simulink model "Multiplier"  (R2019b)
settings: Solver=VariableStepAuto  StartTime=0.0  StopTime=10.0  RelTol=1e-3
libraries: hdlsllib x17
(part 2 of 3)

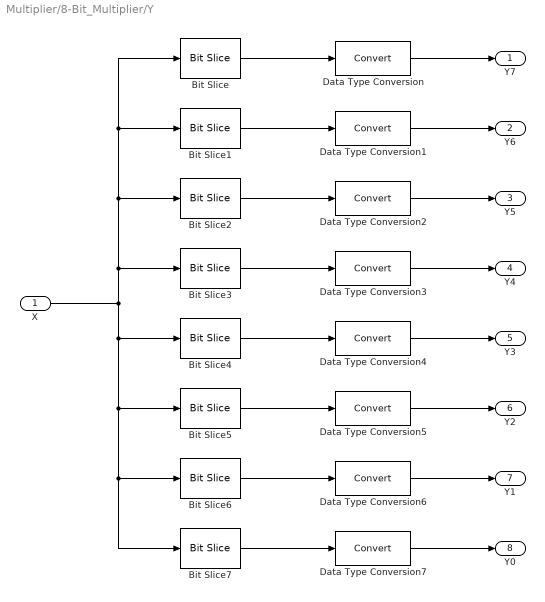
== system Multiplier/8-Bit_Multiplier/Y ==
  X : Inport  OutDataTypeStr=uint8  SampleTime=1
  Bit Slice : hdlsllib/Logic and Bit Operations/Bit Slice  lidx=7  ridx=7
      settings: SourceProductName=Simulink  SourceProductBaseCode=SL
  Bit Slice1 : hdlsllib/Logic and Bit Operations/Bit Slice  lidx=6  ridx=6
      settings: SourceProductName=Simulink  SourceProductBaseCode=SL
  Bit Slice2 : hdlsllib/Logic and Bit Operations/Bit Slice  lidx=5  ridx=5
      settings: SourceProductName=Simulink  SourceProductBaseCode=SL
  Bit Slice3 : hdlsllib/Logic and Bit Operations/Bit Slice  lidx=4  ridx=4
      settings: SourceProductName=Simulink  SourceProductBaseCode=SL
  Bit Slice4 : hdlsllib/Logic and Bit Operations/Bit Slice  lidx=3  ridx=3
      settings: SourceProductName=Simulink  SourceProductBaseCode=SL
  Bit Slice5 : hdlsllib/Logic and Bit Operations/Bit Slice  lidx=2  ridx=2
      settings: SourceProductName=Simulink  SourceProductBaseCode=SL
  Bit Slice6 : hdlsllib/Logic and Bit Operations/Bit Slice  lidx=1  ridx=1
      settings: SourceProductName=Simulink  SourceProductBaseCode=SL
  Bit Slice7 : hdlsllib/Logic and Bit Operations/Bit Slice  lidx=0  ridx=0
      settings: SourceProductName=Simulink  SourceProductBaseCode=SL
  Data Type Conversion{,1..7} (8 alike) : DataTypeConversion
  Y7 : Outport
  Y6 : Outport  Port=2
  Y5 : Outport  Port=3
  Y4 : Outport  Port=4
  Y3 : Outport  Port=5
  Y2 : Outport  Port=6
  Y1 : Outport  Port=7
  Y0 : Outport  Port=8
  wires:
  Bit Slice6/1 -> Data Type Conversion6/1
  X/1 -> Bit Slice3/1, Bit Slice2/1, Bit Slice1/1, Bit Slice/1, Bit Slice4/1, Bit Slice5/1, Bit Slice6/1, Bit Slice7/1
  Bit Slice/1 -> Data Type Conversion/1
  Bit Slice7/1 -> Data Type Conversion7/1
  Bit Slice4/1 -> Data Type Conversion4/1
  Bit Slice1/1 -> Data Type Conversion1/1
  Bit Slice3/1 -> Data Type Conversion3/1
  Data Type Conversion1/1 -> Y6/1
  Data Type Conversion7/1 -> Y0/1
  Data Type Conversion5/1 -> Y2/1
  Data Type Conversion3/1 -> Y4/1
  Data Type Conversion4/1 -> Y3/1
  Bit Slice2/1 -> Data Type Conversion2/1
  Bit Slice5/1 -> Data Type Conversion5/1
  Data Type Conversion6/1 -> Y1/1
  Data Type Conversion/1 -> Y7/1
  Data Type Conversion2/1 -> Y5/1

== system Multiplier/8-Bit_Multiplier/Full adder1/Half adder1 ==
  In1 : Inport  OutDataTypeStr=boolean
  In2 : Inport  Port=2  OutDataTypeStr=boolean
  Logical Operator : Logic  AllPortsSameDT=off  OutDataTypeStr=boolean
  Logical Operator1 : Logic  Operator=XOR  AllPortsSameDT=off  OutDataTypeStr=boolean
  Out1 : Outport
  Out2 : Outport  Port=2
  wires:
  In2/1 -> Logical Operator/2, Logical Operator1/2
  In1/1 -> Logical Operator/1, Logical Operator1/1
  Logical Operator1/1 -> Out1/1
  Logical Operator/1 -> Out2/1

== system Multiplier/8-Bit_Multiplier/Full adder1/Half adder2 ==
  In1 : Inport  OutDataTypeStr=boolean
  In2 : Inport  Port=2  OutDataTypeStr=boolean
  Logical Operator : Logic  AllPortsSameDT=off  OutDataTypeStr=boolean
  Logical Operator1 : Logic  Operator=XOR  AllPortsSameDT=off  OutDataTypeStr=boolean
  Out1 : Outport
  Out2 : Outport  Port=2
  wires:
  In2/1 -> Logical Operator/2, Logical Operator1/2
  In1/1 -> Logical Operator/1, Logical Operator1/1
  Logical Operator1/1 -> Out1/1
  Logical Operator/1 -> Out2/1

== system Multiplier/8-Bit_Multiplier/Full adder10/Half adder1 ==
  In1 : Inport  OutDataTypeStr=boolean
  In2 : Inport  Port=2  OutDataTypeStr=boolean
  Logical Operator : Logic  AllPortsSameDT=off  OutDataTypeStr=boolean
  Logical Operator1 : Logic  Operator=XOR  AllPortsSameDT=off  OutDataTypeStr=boolean
  Out1 : Outport
  Out2 : Outport  Port=2
  wires:
  In2/1 -> Logical Operator/2, Logical Operator1/2
  In1/1 -> Logical Operator/1, Logical Operator1/1
  Logical Operator1/1 -> Out1/1
  Logical Operator/1 -> Out2/1

== system Multiplier/8-Bit_Multiplier/Full adder10/Half adder2 ==
  In1 : Inport  OutDataTypeStr=boolean
  In2 : Inport  Port=2  OutDataTypeStr=boolean
  Logical Operator : Logic  AllPortsSameDT=off  OutDataTypeStr=boolean
  Logical Operator1 : Logic  Operator=XOR  AllPortsSameDT=off  OutDataTypeStr=boolean
  Out1 : Outport
  Out2 : Outport  Port=2
  wires:
  In2/1 -> Logical Operator/2, Logical Operator1/2
  In1/1 -> Logical Operator/1, Logical Operator1/1
  Logical Operator1/1 -> Out1/1
  Logical Operator/1 -> Out2/1

== system Multiplier/8-Bit_Multiplier/Full adder11/Half adder1 ==
  In1 : Inport  OutDataTypeStr=boolean
  In2 : Inport  Port=2  OutDataTypeStr=boolean
  Logical Operator : Logic  AllPortsSameDT=off  OutDataTypeStr=boolean
  Logical Operator1 : Logic  Operator=XOR  AllPortsSameDT=off  OutDataTypeStr=boolean
  Out1 : Outport
  Out2 : Outport  Port=2
  wires:
  In2/1 -> Logical Operator/2, Logical Operator1/2
  In1/1 -> Logical Operator/1, Logical Operator1/1
  Logical Operator1/1 -> Out1/1
  Logical Operator/1 -> Out2/1

== system Multiplier/8-Bit_Multiplier/Full adder11/Half adder2 ==
  In1 : Inport  OutDataTypeStr=boolean
  In2 : Inport  Port=2  OutDataTypeStr=boolean
  Logical Operator : Logic  AllPortsSameDT=off  OutDataTypeStr=boolean
  Logical Operator1 : Logic  Operator=XOR  AllPortsSameDT=off  OutDataTypeStr=boolean
  Out1 : Outport
  Out2 : Outport  Port=2
  wires:
  In2/1 -> Logical Operator/2, Logical Operator1/2
  In1/1 -> Logical Operator/1, Logical Operator1/1
  Logical Operator1/1 -> Out1/1
  Logical Operator/1 -> Out2/1

== system Multiplier/8-Bit_Multiplier/Full adder12/Half adder1 ==
  In1 : Inport  OutDataTypeStr=boolean
  In2 : Inport  Port=2  OutDataTypeStr=boolean
  Logical Operator : Logic  AllPortsSameDT=off  OutDataTypeStr=boolean
  Logical Operator1 : Logic  Operator=XOR  AllPortsSameDT=off  OutDataTypeStr=boolean
  Out1 : Outport
  Out2 : Outport  Port=2
  wires:
  In2/1 -> Logical Operator/2, Logical Operator1/2
  In1/1 -> Logical Operator/1, Logical Operator1/1
  Logical Operator1/1 -> Out1/1
  Logical Operator/1 -> Out2/1

== system Multiplier/8-Bit_Multiplier/Full adder12/Half adder2 ==
  In1 : Inport  OutDataTypeStr=boolean
  In2 : Inport  Port=2  OutDataTypeStr=boolean
  Logical Operator : Logic  AllPortsSameDT=off  OutDataTypeStr=boolean
  Logical Operator1 : Logic  Operator=XOR  AllPortsSameDT=off  OutDataTypeStr=boolean
  Out1 : Outport
  Out2 : Outport  Port=2
  wires:
  In2/1 -> Logical Operator/2, Logical Operator1/2
  In1/1 -> Logical Operator/1, Logical Operator1/1
  Logical Operator1/1 -> Out1/1
  Logical Operator/1 -> Out2/1

== system Multiplier/8-Bit_Multiplier/Full adder13/Half adder1 ==
  In1 : Inport  OutDataTypeStr=boolean
  In2 : Inport  Port=2  OutDataTypeStr=boolean
  Logical Operator : Logic  AllPortsSameDT=off  OutDataTypeStr=boolean
  Logical Operator1 : Logic  Operator=XOR  AllPortsSameDT=off  OutDataTypeStr=boolean
  Out1 : Outport
  Out2 : Outport  Port=2
  wires:
  In2/1 -> Logical Operator/2, Logical Operator1/2
  In1/1 -> Logical Operator/1, Logical Operator1/1
  Logical Operator1/1 -> Out1/1
  Logical Operator/1 -> Out2/1

== system Multiplier/8-Bit_Multiplier/Full adder13/Half adder2 ==
  In1 : Inport  OutDataTypeStr=boolean
  In2 : Inport  Port=2  OutDataTypeStr=boolean
  Logical Operator : Logic  AllPortsSameDT=off  OutDataTypeStr=boolean
  Logical Operator1 : Logic  Operator=XOR  AllPortsSameDT=off  OutDataTypeStr=boolean
  Out1 : Outport
  Out2 : Outport  Port=2
  wires:
  In2/1 -> Logical Operator/2, Logical Operator1/2
  In1/1 -> Logical Operator/1, Logical Operator1/1
  Logical Operator1/1 -> Out1/1
  Logical Operator/1 -> Out2/1

== system Multiplier/8-Bit_Multiplier/Full adder14/Half adder1 ==
  In1 : Inport  OutDataTypeStr=boolean
  In2 : Inport  Port=2  OutDataTypeStr=boolean
  Logical Operator : Logic  AllPortsSameDT=off  OutDataTypeStr=boolean
  Logical Operator1 : Logic  Operator=XOR  AllPortsSameDT=off  OutDataTypeStr=boolean
  Out1 : Outport
  Out2 : Outport  Port=2
  wires:
  In2/1 -> Logical Operator/2, Logical Operator1/2
  In1/1 -> Logical Operator/1, Logical Operator1/1
  Logical Operator1/1 -> Out1/1
  Logical Operator/1 -> Out2/1

== system Multiplier/8-Bit_Multiplier/Full adder14/Half adder2 ==
  In1 : Inport  OutDataTypeStr=boolean
  In2 : Inport  Port=2  OutDataTypeStr=boolean
  Logical Operator : Logic  AllPortsSameDT=off  OutDataTypeStr=boolean
  Logical Operator1 : Logic  Operator=XOR  AllPortsSameDT=off  OutDataTypeStr=boolean
  Out1 : Outport
  Out2 : Outport  Port=2
  wires:
  In2/1 -> Logical Operator/2, Logical Operator1/2
  In1/1 -> Logical Operator/1, Logical Operator1/1
  Logical Operator1/1 -> Out1/1
  Logical Operator/1 -> Out2/1

== system Multiplier/8-Bit_Multiplier/Full adder15/Half adder1 ==
  In1 : Inport  OutDataTypeStr=boolean
  In2 : Inport  Port=2  OutDataTypeStr=boolean
  Logical Operator : Logic  AllPortsSameDT=off  OutDataTypeStr=boolean
  Logical Operator1 : Logic  Operator=XOR  AllPortsSameDT=off  OutDataTypeStr=boolean
  Out1 : Outport
  Out2 : Outport  Port=2
  wires:
  In2/1 -> Logical Operator/2, Logical Operator1/2
  In1/1 -> Logical Operator/1, Logical Operator1/1
  Logical Operator1/1 -> Out1/1
  Logical Operator/1 -> Out2/1

== system Multiplier/8-Bit_Multiplier/Full adder15/Half adder2 ==
  In1 : Inport  OutDataTypeStr=boolean
  In2 : Inport  Port=2  OutDataTypeStr=boolean
  Logical Operator : Logic  AllPortsSameDT=off  OutDataTypeStr=boolean
  Logical Operator1 : Logic  Operator=XOR  AllPortsSameDT=off  OutDataTypeStr=boolean
  Out1 : Outport
  Out2 : Outport  Port=2
  wires:
  In2/1 -> Logical Operator/2, Logical Operator1/2
  In1/1 -> Logical Operator/1, Logical Operator1/1
  Logical Operator1/1 -> Out1/1
  Logical Operator/1 -> Out2/1

== system Multiplier/8-Bit_Multiplier/Full adder16/Half adder1 ==
  In1 : Inport  OutDataTypeStr=boolean
  In2 : Inport  Port=2  OutDataTypeStr=boolean
  Logical Operator : Logic  AllPortsSameDT=off  OutDataTypeStr=boolean
  Logical Operator1 : Logic  Operator=XOR  AllPortsSameDT=off  OutDataTypeStr=boolean
  Out1 : Outport
  Out2 : Outport  Port=2
  wires:
  In2/1 -> Logical Operator/2, Logical Operator1/2
  In1/1 -> Logical Operator/1, Logical Operator1/1
  Logical Operator1/1 -> Out1/1
  Logical Operator/1 -> Out2/1

== system Multiplier/8-Bit_Multiplier/Full adder16/Half adder2 ==
  In1 : Inport  OutDataTypeStr=boolean
  In2 : Inport  Port=2  OutDataTypeStr=boolean
  Logical Operator : Logic  AllPortsSameDT=off  OutDataTypeStr=boolean
  Logical Operator1 : Logic  Operator=XOR  AllPortsSameDT=off  OutDataTypeStr=boolean
  Out1 : Outport
  Out2 : Outport  Port=2
  wires:
  In2/1 -> Logical Operator/2, Logical Operator1/2
  In1/1 -> Logical Operator/1, Logical Operator1/1
  Logical Operator1/1 -> Out1/1
  Logical Operator/1 -> Out2/1

== system Multiplier/8-Bit_Multiplier/Full adder17/Half adder1 ==
  In1 : Inport  OutDataTypeStr=boolean
  In2 : Inport  Port=2  OutDataTypeStr=boolean
  Logical Operator : Logic  AllPortsSameDT=off  OutDataTypeStr=boolean
  Logical Operator1 : Logic  Operator=XOR  AllPortsSameDT=off  OutDataTypeStr=boolean
  Out1 : Outport
  Out2 : Outport  Port=2
  wires:
  In2/1 -> Logical Operator/2, Logical Operator1/2
  In1/1 -> Logical Operator/1, Logical Operator1/1
  Logical Operator1/1 -> Out1/1
  Logical Operator/1 -> Out2/1

== system Multiplier/8-Bit_Multiplier/Full adder17/Half adder2 ==
  In1 : Inport  OutDataTypeStr=boolean
  In2 : Inport  Port=2  OutDataTypeStr=boolean
  Logical Operator : Logic  AllPortsSameDT=off  OutDataTypeStr=boolean
  Logical Operator1 : Logic  Operator=XOR  AllPortsSameDT=off  OutDataTypeStr=boolean
  Out1 : Outport
  Out2 : Outport  Port=2
  wires:
  In2/1 -> Logical Operator/2, Logical Operator1/2
  In1/1 -> Logical Operator/1, Logical Operator1/1
  Logical Operator1/1 -> Out1/1
  Logical Operator/1 -> Out2/1

== system Multiplier/8-Bit_Multiplier/Full adder18/Half adder1 ==
  In1 : Inport  OutDataTypeStr=boolean
  In2 : Inport  Port=2  OutDataTypeStr=boolean
  Logical Operator : Logic  AllPortsSameDT=off  OutDataTypeStr=boolean
  Logical Operator1 : Logic  Operator=XOR  AllPortsSameDT=off  OutDataTypeStr=boolean
  Out1 : Outport
  Out2 : Outport  Port=2
  wires:
  In2/1 -> Logical Operator/2, Logical Operator1/2
  In1/1 -> Logical Operator/1, Logical Operator1/1
  Logical Operator1/1 -> Out1/1
  Logical Operator/1 -> Out2/1

== system Multiplier/8-Bit_Multiplier/Full adder18/Half adder2 ==
  In1 : Inport  OutDataTypeStr=boolean
  In2 : Inport  Port=2  OutDataTypeStr=boolean
  Logical Operator : Logic  AllPortsSameDT=off  OutDataTypeStr=boolean
  Logical Operator1 : Logic  Operator=XOR  AllPortsSameDT=off  OutDataTypeStr=boolean
  Out1 : Outport
  Out2 : Outport  Port=2
  wires:
  In2/1 -> Logical Operator/2, Logical Operator1/2
  In1/1 -> Logical Operator/1, Logical Operator1/1
  Logical Operator1/1 -> Out1/1
  Logical Operator/1 -> Out2/1

== system Multiplier/8-Bit_Multiplier/Full adder19/Half adder1 ==
  In1 : Inport  OutDataTypeStr=boolean
  In2 : Inport  Port=2  OutDataTypeStr=boolean
  Logical Operator : Logic  AllPortsSameDT=off  OutDataTypeStr=boolean
  Logical Operator1 : Logic  Operator=XOR  AllPortsSameDT=off  OutDataTypeStr=boolean
  Out1 : Outport
  Out2 : Outport  Port=2
  wires:
  In2/1 -> Logical Operator/2, Logical Operator1/2
  In1/1 -> Logical Operator/1, Logical Operator1/1
  Logical Operator1/1 -> Out1/1
  Logical Operator/1 -> Out2/1

== system Multiplier/8-Bit_Multiplier/Full adder19/Half adder2 ==
  In1 : Inport  OutDataTypeStr=boolean
  In2 : Inport  Port=2  OutDataTypeStr=boolean
  Logical Operator : Logic  AllPortsSameDT=off  OutDataTypeStr=boolean
  Logical Operator1 : Logic  Operator=XOR  AllPortsSameDT=off  OutDataTypeStr=boolean
  Out1 : Outport
  Out2 : Outport  Port=2
  wires:
  In2/1 -> Logical Operator/2, Logical Operator1/2
  In1/1 -> Logical Operator/1, Logical Operator1/1
  Logical Operator1/1 -> Out1/1
  Logical Operator/1 -> Out2/1

== system Multiplier/8-Bit_Multiplier/Full adder2/Half adder1 ==
  In1 : Inport  OutDataTypeStr=boolean
  In2 : Inport  Port=2  OutDataTypeStr=boolean
  Logical Operator : Logic  AllPortsSameDT=off  OutDataTypeStr=boolean
  Logical Operator1 : Logic  Operator=XOR  AllPortsSameDT=off  OutDataTypeStr=boolean
  Out1 : Outport
  Out2 : Outport  Port=2
  wires:
  In2/1 -> Logical Operator/2, Logical Operator1/2
  In1/1 -> Logical Operator/1, Logical Operator1/1
  Logical Operator1/1 -> Out1/1
  Logical Operator/1 -> Out2/1

== system Multiplier/8-Bit_Multiplier/Full adder2/Half adder2 ==
  In1 : Inport  OutDataTypeStr=boolean
  In2 : Inport  Port=2  OutDataTypeStr=boolean
  Logical Operator : Logic  AllPortsSameDT=off  OutDataTypeStr=boolean
  Logical Operator1 : Logic  Operator=XOR  AllPortsSameDT=off  OutDataTypeStr=boolean
  Out1 : Outport
  Out2 : Outport  Port=2
  wires:
  In2/1 -> Logical Operator/2, Logical Operator1/2
  In1/1 -> Logical Operator/1, Logical Operator1/1
  Logical Operator1/1 -> Out1/1
  Logical Operator/1 -> Out2/1

== system Multiplier/8-Bit_Multiplier/Full adder20/Half adder1 ==
  In1 : Inport  OutDataTypeStr=boolean
  In2 : Inport  Port=2  OutDataTypeStr=boolean
  Logical Operator : Logic  AllPortsSameDT=off  OutDataTypeStr=boolean
  Logical Operator1 : Logic  Operator=XOR  AllPortsSameDT=off  OutDataTypeStr=boolean
  Out1 : Outport
  Out2 : Outport  Port=2
  wires:
  In2/1 -> Logical Operator/2, Logical Operator1/2
  In1/1 -> Logical Operator/1, Logical Operator1/1
  Logical Operator1/1 -> Out1/1
  Logical Operator/1 -> Out2/1

== system Multiplier/8-Bit_Multiplier/Full adder20/Half adder2 ==
  In1 : Inport  OutDataTypeStr=boolean
  In2 : Inport  Port=2  OutDataTypeStr=boolean
  Logical Operator : Logic  AllPortsSameDT=off  OutDataTypeStr=boolean
  Logical Operator1 : Logic  Operator=XOR  AllPortsSameDT=off  OutDataTypeStr=boolean
  Out1 : Outport
  Out2 : Outport  Port=2
  wires:
  In2/1 -> Logical Operator/2, Logical Operator1/2
  In1/1 -> Logical Operator/1, Logical Operator1/1
  Logical Operator1/1 -> Out1/1
  Logical Operator/1 -> Out2/1

== system Multiplier/8-Bit_Multiplier/Full adder21/Half adder1 ==
  In1 : Inport  OutDataTypeStr=boolean
  In2 : Inport  Port=2  OutDataTypeStr=boolean
  Logical Operator : Logic  AllPortsSameDT=off  OutDataTypeStr=boolean
  Logical Operator1 : Logic  Operator=XOR  AllPortsSameDT=off  OutDataTypeStr=boolean
  Out1 : Outport
  Out2 : Outport  Port=2
  wires:
  In2/1 -> Logical Operator/2, Logical Operator1/2
  In1/1 -> Logical Operator/1, Logical Operator1/1
  Logical Operator1/1 -> Out1/1
  Logical Operator/1 -> Out2/1

== system Multiplier/8-Bit_Multiplier/Full adder21/Half adder2 ==
  In1 : Inport  OutDataTypeStr=boolean
  In2 : Inport  Port=2  OutDataTypeStr=boolean
  Logical Operator : Logic  AllPortsSameDT=off  OutDataTypeStr=boolean
  Logical Operator1 : Logic  Operator=XOR  AllPortsSameDT=off  OutDataTypeStr=boolean
  Out1 : Outport
  Out2 : Outport  Port=2
  wires:
  In2/1 -> Logical Operator/2, Logical Operator1/2
  In1/1 -> Logical Operator/1, Logical Operator1/1
  Logical Operator1/1 -> Out1/1
  Logical Operator/1 -> Out2/1

== system Multiplier/8-Bit_Multiplier/Full adder22/Half adder1 ==
  In1 : Inport  OutDataTypeStr=boolean
  In2 : Inport  Port=2  OutDataTypeStr=boolean
  Logical Operator : Logic  AllPortsSameDT=off  OutDataTypeStr=boolean
  Logical Operator1 : Logic  Operator=XOR  AllPortsSameDT=off  OutDataTypeStr=boolean
  Out1 : Outport
  Out2 : Outport  Port=2
  wires:
  In2/1 -> Logical Operator/2, Logical Operator1/2
  In1/1 -> Logical Operator/1, Logical Operator1/1
  Logical Operator1/1 -> Out1/1
  Logical Operator/1 -> Out2/1

== system Multiplier/8-Bit_Multiplier/Full adder22/Half adder2 ==
  In1 : Inport  OutDataTypeStr=boolean
  In2 : Inport  Port=2  OutDataTypeStr=boolean
  Logical Operator : Logic  AllPortsSameDT=off  OutDataTypeStr=boolean
  Logical Operator1 : Logic  Operator=XOR  AllPortsSameDT=off  OutDataTypeStr=boolean
  Out1 : Outport
  Out2 : Outport  Port=2
  wires:
  In2/1 -> Logical Operator/2, Logical Operator1/2
  In1/1 -> Logical Operator/1, Logical Operator1/1
  Logical Operator1/1 -> Out1/1
  Logical Operator/1 -> Out2/1

== system Multiplier/8-Bit_Multiplier/Full adder23/Half adder1 ==
  In1 : Inport  OutDataTypeStr=boolean
  In2 : Inport  Port=2  OutDataTypeStr=boolean
  Logical Operator : Logic  AllPortsSameDT=off  OutDataTypeStr=boolean
  Logical Operator1 : Logic  Operator=XOR  AllPortsSameDT=off  OutDataTypeStr=boolean
  Out1 : Outport
  Out2 : Outport  Port=2
  wires:
  In2/1 -> Logical Operator/2, Logical Operator1/2
  In1/1 -> Logical Operator/1, Logical Operator1/1
  Logical Operator1/1 -> Out1/1
  Logical Operator/1 -> Out2/1

== system Multiplier/8-Bit_Multiplier/Full adder23/Half adder2 ==
  In1 : Inport  OutDataTypeStr=boolean
  In2 : Inport  Port=2  OutDataTypeStr=boolean
  Logical Operator : Logic  AllPortsSameDT=off  OutDataTypeStr=boolean
  Logical Operator1 : Logic  Operator=XOR  AllPortsSameDT=off  OutDataTypeStr=boolean
  Out1 : Outport
  Out2 : Outport  Port=2
  wires:
  In2/1 -> Logical Operator/2, Logical Operator1/2
  In1/1 -> Logical Operator/1, Logical Operator1/1
  Logical Operator1/1 -> Out1/1
  Logical Operator/1 -> Out2/1

== system Multiplier/8-Bit_Multiplier/Full adder24/Half adder1 ==
  In1 : Inport  OutDataTypeStr=boolean
  In2 : Inport  Port=2  OutDataTypeStr=boolean
  Logical Operator : Logic  AllPortsSameDT=off  OutDataTypeStr=boolean
  Logical Operator1 : Logic  Operator=XOR  AllPortsSameDT=off  OutDataTypeStr=boolean
  Out1 : Outport
  Out2 : Outport  Port=2
  wires:
  In2/1 -> Logical Operator/2, Logical Operator1/2
  In1/1 -> Logical Operator/1, Logical Operator1/1
  Logical Operator1/1 -> Out1/1
  Logical Operator/1 -> Out2/1

== system Multiplier/8-Bit_Multiplier/Full adder24/Half adder2 ==
  In1 : Inport  OutDataTypeStr=boolean
  In2 : Inport  Port=2  OutDataTypeStr=boolean
  Logical Operator : Logic  AllPortsSameDT=off  OutDataTypeStr=boolean
  Logical Operator1 : Logic  Operator=XOR  AllPortsSameDT=off  OutDataTypeStr=boolean
  Out1 : Outport
  Out2 : Outport  Port=2
  wires:
  In2/1 -> Logical Operator/2, Logical Operator1/2
  In1/1 -> Logical Operator/1, Logical Operator1/1
  Logical Operator1/1 -> Out1/1
  Logical Operator/1 -> Out2/1

== system Multiplier/8-Bit_Multiplier/Full adder25/Half adder1 ==
  In1 : Inport  OutDataTypeStr=boolean
  In2 : Inport  Port=2  OutDataTypeStr=boolean
  Logical Operator : Logic  AllPortsSameDT=off  OutDataTypeStr=boolean
  Logical Operator1 : Logic  Operator=XOR  AllPortsSameDT=off  OutDataTypeStr=boolean
  Out1 : Outport
  Out2 : Outport  Port=2
  wires:
  In2/1 -> Logical Operator/2, Logical Operator1/2
  In1/1 -> Logical Operator/1, Logical Operator1/1
  Logical Operator1/1 -> Out1/1
  Logical Operator/1 -> Out2/1

== system Multiplier/8-Bit_Multiplier/Full adder25/Half adder2 ==
  In1 : Inport  OutDataTypeStr=boolean
  In2 : Inport  Port=2  OutDataTypeStr=boolean
  Logical Operator : Logic  AllPortsSameDT=off  OutDataTypeStr=boolean
  Logical Operator1 : Logic  Operator=XOR  AllPortsSameDT=off  OutDataTypeStr=boolean
  Out1 : Outport
  Out2 : Outport  Port=2
  wires:
  In2/1 -> Logical Operator/2, Logical Operator1/2
  In1/1 -> Logical Operator/1, Logical Operator1/1
  Logical Operator1/1 -> Out1/1
  Logical Operator/1 -> Out2/1

== system Multiplier/8-Bit_Multiplier/Full adder26/Half adder1 ==
  In1 : Inport  OutDataTypeStr=boolean
  In2 : Inport  Port=2  OutDataTypeStr=boolean
  Logical Operator : Logic  AllPortsSameDT=off  OutDataTypeStr=boolean
  Logical Operator1 : Logic  Operator=XOR  AllPortsSameDT=off  OutDataTypeStr=boolean
  Out1 : Outport
  Out2 : Outport  Port=2
  wires:
  In2/1 -> Logical Operator/2, Logical Operator1/2
  In1/1 -> Logical Operator/1, Logical Operator1/1
  Logical Operator1/1 -> Out1/1
  Logical Operator/1 -> Out2/1

== system Multiplier/8-Bit_Multiplier/Full adder26/Half adder2 ==
  In1 : Inport  OutDataTypeStr=boolean
  In2 : Inport  Port=2  OutDataTypeStr=boolean
  Logical Operator : Logic  AllPortsSameDT=off  OutDataTypeStr=boolean
  Logical Operator1 : Logic  Operator=XOR  AllPortsSameDT=off  OutDataTypeStr=boolean
  Out1 : Outport
  Out2 : Outport  Port=2
  wires:
  In2/1 -> Logical Operator/2, Logical Operator1/2
  In1/1 -> Logical Operator/1, Logical Operator1/1
  Logical Operator1/1 -> Out1/1
  Logical Operator/1 -> Out2/1

== system Multiplier/8-Bit_Multiplier/Full adder27/Half adder1 ==
  In1 : Inport  OutDataTypeStr=boolean
  In2 : Inport  Port=2  OutDataTypeStr=boolean
  Logical Operator : Logic  AllPortsSameDT=off  OutDataTypeStr=boolean
  Logical Operator1 : Logic  Operator=XOR  AllPortsSameDT=off  OutDataTypeStr=boolean
  Out1 : Outport
  Out2 : Outport  Port=2
  wires:
  In2/1 -> Logical Operator/2, Logical Operator1/2
  In1/1 -> Logical Operator/1, Logical Operator1/1
  Logical Operator1/1 -> Out1/1
  Logical Operator/1 -> Out2/1

== system Multiplier/8-Bit_Multiplier/Full adder27/Half adder2 ==
  In1 : Inport  OutDataTypeStr=boolean
  In2 : Inport  Port=2  OutDataTypeStr=boolean
  Logical Operator : Logic  AllPortsSameDT=off  OutDataTypeStr=boolean
  Logical Operator1 : Logic  Operator=XOR  AllPortsSameDT=off  OutDataTypeStr=boolean
  Out1 : Outport
  Out2 : Outport  Port=2
  wires:
  In2/1 -> Logical Operator/2, Logical Operator1/2
  In1/1 -> Logical Operator/1, Logical Operator1/1
  Logical Operator1/1 -> Out1/1
  Logical Operator/1 -> Out2/1

== system Multiplier/8-Bit_Multiplier/Full adder28/Half adder1 ==
  In1 : Inport  OutDataTypeStr=boolean
  In2 : Inport  Port=2  OutDataTypeStr=boolean
  Logical Operator : Logic  AllPortsSameDT=off  OutDataTypeStr=boolean
  Logical Operator1 : Logic  Operator=XOR  AllPortsSameDT=off  OutDataTypeStr=boolean
  Out1 : Outport
  Out2 : Outport  Port=2
  wires:
  In2/1 -> Logical Operator/2, Logical Operator1/2
  In1/1 -> Logical Operator/1, Logical Operator1/1
  Logical Operator1/1 -> Out1/1
  Logical Operator/1 -> Out2/1

== system Multiplier/8-Bit_Multiplier/Full adder28/Half adder2 ==
  In1 : Inport  OutDataTypeStr=boolean
  In2 : Inport  Port=2  OutDataTypeStr=boolean
  Logical Operator : Logic  AllPortsSameDT=off  OutDataTypeStr=boolean
  Logical Operator1 : Logic  Operator=XOR  AllPortsSameDT=off  OutDataTypeStr=boolean
  Out1 : Outport
  Out2 : Outport  Port=2
  wires:
  In2/1 -> Logical Operator/2, Logical Operator1/2
  In1/1 -> Logical Operator/1, Logical Operator1/1
  Logical Operator1/1 -> Out1/1
  Logical Operator/1 -> Out2/1

== system Multiplier/8-Bit_Multiplier/Full adder29/Half adder1 ==
  In1 : Inport  OutDataTypeStr=boolean
  In2 : Inport  Port=2  OutDataTypeStr=boolean
  Logical Operator : Logic  AllPortsSameDT=off  OutDataTypeStr=boolean
  Logical Operator1 : Logic  Operator=XOR  AllPortsSameDT=off  OutDataTypeStr=boolean
  Out1 : Outport
  Out2 : Outport  Port=2
  wires:
  In2/1 -> Logical Operator/2, Logical Operator1/2
  In1/1 -> Logical Operator/1, Logical Operator1/1
  Logical Operator1/1 -> Out1/1
  Logical Operator/1 -> Out2/1

== system Multiplier/8-Bit_Multiplier/Full adder29/Half adder2 ==
  In1 : Inport  OutDataTypeStr=boolean
  In2 : Inport  Port=2  OutDataTypeStr=boolean
  Logical Operator : Logic  AllPortsSameDT=off  OutDataTypeStr=boolean
  Logical Operator1 : Logic  Operator=XOR  AllPortsSameDT=off  OutDataTypeStr=boolean
  Out1 : Outport
  Out2 : Outport  Port=2
  wires:
  In2/1 -> Logical Operator/2, Logical Operator1/2
  In1/1 -> Logical Operator/1, Logical Operator1/1
  Logical Operator1/1 -> Out1/1
  Logical Operator/1 -> Out2/1

== system Multiplier/8-Bit_Multiplier/Full adder3/Half adder1 ==
  In1 : Inport  OutDataTypeStr=boolean
  In2 : Inport  Port=2  OutDataTypeStr=boolean
  Logical Operator : Logic  AllPortsSameDT=off  OutDataTypeStr=boolean
  Logical Operator1 : Logic  Operator=XOR  AllPortsSameDT=off  OutDataTypeStr=boolean
  Out1 : Outport
  Out2 : Outport  Port=2
  wires:
  In2/1 -> Logical Operator/2, Logical Operator1/2
  In1/1 -> Logical Operator/1, Logical Operator1/1
  Logical Operator1/1 -> Out1/1
  Logical Operator/1 -> Out2/1

== system Multiplier/8-Bit_Multiplier/Full adder3/Half adder2 ==
  In1 : Inport  OutDataTypeStr=boolean
  In2 : Inport  Port=2  OutDataTypeStr=boolean
  Logical Operator : Logic  AllPortsSameDT=off  OutDataTypeStr=boolean
  Logical Operator1 : Logic  Operator=XOR  AllPortsSameDT=off  OutDataTypeStr=boolean
  Out1 : Outport
  Out2 : Outport  Port=2
  wires:
  In2/1 -> Logical Operator/2, Logical Operator1/2
  In1/1 -> Logical Operator/1, Logical Operator1/1
  Logical Operator1/1 -> Out1/1
  Logical Operator/1 -> Out2/1

== system Multiplier/8-Bit_Multiplier/Full adder30/Half adder1 ==
  In1 : Inport  OutDataTypeStr=boolean
  In2 : Inport  Port=2  OutDataTypeStr=boolean
  Logical Operator : Logic  AllPortsSameDT=off  OutDataTypeStr=boolean
  Logical Operator1 : Logic  Operator=XOR  AllPortsSameDT=off  OutDataTypeStr=boolean
  Out1 : Outport
  Out2 : Outport  Port=2
  wires:
  In2/1 -> Logical Operator/2, Logical Operator1/2
  In1/1 -> Logical Operator/1, Logical Operator1/1
  Logical Operator1/1 -> Out1/1
  Logical Operator/1 -> Out2/1

== system Multiplier/8-Bit_Multiplier/Full adder30/Half adder2 ==
  In1 : Inport  OutDataTypeStr=boolean
  In2 : Inport  Port=2  OutDataTypeStr=boolean
  Logical Operator : Logic  AllPortsSameDT=off  OutDataTypeStr=boolean
  Logical Operator1 : Logic  Operator=XOR  AllPortsSameDT=off  OutDataTypeStr=boolean
  Out1 : Outport
  Out2 : Outport  Port=2
  wires:
  In2/1 -> Logical Operator/2, Logical Operator1/2
  In1/1 -> Logical Operator/1, Logical Operator1/1
  Logical Operator1/1 -> Out1/1
  Logical Operator/1 -> Out2/1

== system Multiplier/8-Bit_Multiplier/Full adder31/Half adder1 ==
  In1 : Inport  OutDataTypeStr=boolean
  In2 : Inport  Port=2  OutDataTypeStr=boolean
  Logical Operator : Logic  AllPortsSameDT=off  OutDataTypeStr=boolean
  Logical Operator1 : Logic  Operator=XOR  AllPortsSameDT=off  OutDataTypeStr=boolean
  Out1 : Outport
  Out2 : Outport  Port=2
  wires:
  In2/1 -> Logical Operator/2, Logical Operator1/2
  In1/1 -> Logical Operator/1, Logical Operator1/1
  Logical Operator1/1 -> Out1/1
  Logical Operator/1 -> Out2/1

== system Multiplier/8-Bit_Multiplier/Full adder31/Half adder2 ==
  In1 : Inport  OutDataTypeStr=boolean
  In2 : Inport  Port=2  OutDataTypeStr=boolean
  Logical Operator : Logic  AllPortsSameDT=off  OutDataTypeStr=boolean
  Logical Operator1 : Logic  Operator=XOR  AllPortsSameDT=off  OutDataTypeStr=boolean
  Out1 : Outport
  Out2 : Outport  Port=2
  wires:
  In2/1 -> Logical Operator/2, Logical Operator1/2
  In1/1 -> Logical Operator/1, Logical Operator1/1
  Logical Operator1/1 -> Out1/1
  Logical Operator/1 -> Out2/1

== system Multiplier/8-Bit_Multiplier/Full adder32/Half adder1 ==
  In1 : Inport  OutDataTypeStr=boolean
  In2 : Inport  Port=2  OutDataTypeStr=boolean
  Logical Operator : Logic  AllPortsSameDT=off  OutDataTypeStr=boolean
  Logical Operator1 : Logic  Operator=XOR  AllPortsSameDT=off  OutDataTypeStr=boolean
  Out1 : Outport
  Out2 : Outport  Port=2
  wires:
  In2/1 -> Logical Operator/2, Logical Operator1/2
  In1/1 -> Logical Operator/1, Logical Operator1/1
  Logical Operator1/1 -> Out1/1
  Logical Operator/1 -> Out2/1

== system Multiplier/8-Bit_Multiplier/Full adder32/Half adder2 ==
  In1 : Inport  OutDataTypeStr=boolean
  In2 : Inport  Port=2  OutDataTypeStr=boolean
  Logical Operator : Logic  AllPortsSameDT=off  OutDataTypeStr=boolean
  Logical Operator1 : Logic  Operator=XOR  AllPortsSameDT=off  OutDataTypeStr=boolean
  Out1 : Outport
  Out2 : Outport  Port=2
  wires:
  In2/1 -> Logical Operator/2, Logical Operator1/2
  In1/1 -> Logical Operator/1, Logical Operator1/1
  Logical Operator1/1 -> Out1/1
  Logical Operator/1 -> Out2/1

== system Multiplier/8-Bit_Multiplier/Full adder33/Half adder1 ==
  In1 : Inport  OutDataTypeStr=boolean
  In2 : Inport  Port=2  OutDataTypeStr=boolean
  Logical Operator : Logic  AllPortsSameDT=off  OutDataTypeStr=boolean
  Logical Operator1 : Logic  Operator=XOR  AllPortsSameDT=off  OutDataTypeStr=boolean
  Out1 : Outport
  Out2 : Outport  Port=2
  wires:
  In2/1 -> Logical Operator/2, Logical Operator1/2
  In1/1 -> Logical Operator/1, Logical Operator1/1
  Logical Operator1/1 -> Out1/1
  Logical Operator/1 -> Out2/1

== system Multiplier/8-Bit_Multiplier/Full adder33/Half adder2 ==
  In1 : Inport  OutDataTypeStr=boolean
  In2 : Inport  Port=2  OutDataTypeStr=boolean
  Logical Operator : Logic  AllPortsSameDT=off  OutDataTypeStr=boolean
  Logical Operator1 : Logic  Operator=XOR  AllPortsSameDT=off  OutDataTypeStr=boolean
  Out1 : Outport
  Out2 : Outport  Port=2
  wires:
  In2/1 -> Logical Operator/2, Logical Operator1/2
  In1/1 -> Logical Operator/1, Logical Operator1/1
  Logical Operator1/1 -> Out1/1
  Logical Operator/1 -> Out2/1

== system Multiplier/8-Bit_Multiplier/Full adder34/Half adder1 ==
  In1 : Inport  OutDataTypeStr=boolean
  In2 : Inport  Port=2  OutDataTypeStr=boolean
  Logical Operator : Logic  AllPortsSameDT=off  OutDataTypeStr=boolean
  Logical Operator1 : Logic  Operator=XOR  AllPortsSameDT=off  OutDataTypeStr=boolean
  Out1 : Outport
  Out2 : Outport  Port=2
  wires:
  In2/1 -> Logical Operator/2, Logical Operator1/2
  In1/1 -> Logical Operator/1, Logical Operator1/1
  Logical Operator1/1 -> Out1/1
  Logical Operator/1 -> Out2/1

== system Multiplier/8-Bit_Multiplier/Full adder34/Half adder2 ==
  In1 : Inport  OutDataTypeStr=boolean
  In2 : Inport  Port=2  OutDataTypeStr=boolean
  Logical Operator : Logic  AllPortsSameDT=off  OutDataTypeStr=boolean
  Logical Operator1 : Logic  Operator=XOR  AllPortsSameDT=off  OutDataTypeStr=boolean
  Out1 : Outport
  Out2 : Outport  Port=2
  wires:
  In2/1 -> Logical Operator/2, Logical Operator1/2
  In1/1 -> Logical Operator/1, Logical Operator1/1
  Logical Operator1/1 -> Out1/1
  Logical Operator/1 -> Out2/1

== system Multiplier/8-Bit_Multiplier/Full adder35/Half adder1 ==
  In1 : Inport  OutDataTypeStr=boolean
  In2 : Inport  Port=2  OutDataTypeStr=boolean
  Logical Operator : Logic  AllPortsSameDT=off  OutDataTypeStr=boolean
  Logical Operator1 : Logic  Operator=XOR  AllPortsSameDT=off  OutDataTypeStr=boolean
  Out1 : Outport
  Out2 : Outport  Port=2
  wires:
  In2/1 -> Logical Operator/2, Logical Operator1/2
  In1/1 -> Logical Operator/1, Logical Operator1/1
  Logical Operator1/1 -> Out1/1
  Logical Operator/1 -> Out2/1

== system Multiplier/8-Bit_Multiplier/Full adder35/Half adder2 ==
  In1 : Inport  OutDataTypeStr=boolean
  In2 : Inport  Port=2  OutDataTypeStr=boolean
  Logical Operator : Logic  AllPortsSameDT=off  OutDataTypeStr=boolean
  Logical Operator1 : Logic  Operator=XOR  AllPortsSameDT=off  OutDataTypeStr=boolean
  Out1 : Outport
  Out2 : Outport  Port=2
  wires:
  In2/1 -> Logical Operator/2, Logical Operator1/2
  In1/1 -> Logical Operator/1, Logical Operator1/1
  Logical Operator1/1 -> Out1/1
  Logical Operator/1 -> Out2/1

== system Multiplier/8-Bit_Multiplier/Full adder36/Half adder1 ==
  In1 : Inport  OutDataTypeStr=boolean
  In2 : Inport  Port=2  OutDataTypeStr=boolean
  Logical Operator : Logic  AllPortsSameDT=off  OutDataTypeStr=boolean
  Logical Operator1 : Logic  Operator=XOR  AllPortsSameDT=off  OutDataTypeStr=boolean
  Out1 : Outport
  Out2 : Outport  Port=2
  wires:
  In2/1 -> Logical Operator/2, Logical Operator1/2
  In1/1 -> Logical Operator/1, Logical Operator1/1
  Logical Operator1/1 -> Out1/1
  Logical Operator/1 -> Out2/1

== system Multiplier/8-Bit_Multiplier/Full adder36/Half adder2 ==
  In1 : Inport  OutDataTypeStr=boolean
  In2 : Inport  Port=2  OutDataTypeStr=boolean
  Logical Operator : Logic  AllPortsSameDT=off  OutDataTypeStr=boolean
  Logical Operator1 : Logic  Operator=XOR  AllPortsSameDT=off  OutDataTypeStr=boolean
  Out1 : Outport
  Out2 : Outport  Port=2
  wires:
  In2/1 -> Logical Operator/2, Logical Operator1/2
  In1/1 -> Logical Operator/1, Logical Operator1/1
  Logical Operator1/1 -> Out1/1
  Logical Operator/1 -> Out2/1

== system Multiplier/8-Bit_Multiplier/Full adder37/Half adder1 ==
  In1 : Inport  OutDataTypeStr=boolean
  In2 : Inport  Port=2  OutDataTypeStr=boolean
  Logical Operator : Logic  AllPortsSameDT=off  OutDataTypeStr=boolean
  Logical Operator1 : Logic  Operator=XOR  AllPortsSameDT=off  OutDataTypeStr=boolean
  Out1 : Outport
  Out2 : Outport  Port=2
  wires:
  In2/1 -> Logical Operator/2, Logical Operator1/2
  In1/1 -> Logical Operator/1, Logical Operator1/1
  Logical Operator1/1 -> Out1/1
  Logical Operator/1 -> Out2/1

== system Multiplier/8-Bit_Multiplier/Full adder37/Half adder2 ==
  In1 : Inport  OutDataTypeStr=boolean
  In2 : Inport  Port=2  OutDataTypeStr=boolean
  Logical Operator : Logic  AllPortsSameDT=off  OutDataTypeStr=boolean
  Logical Operator1 : Logic  Operator=XOR  AllPortsSameDT=off  OutDataTypeStr=boolean
  Out1 : Outport
  Out2 : Outport  Port=2
  wires:
  In2/1 -> Logical Operator/2, Logical Operator1/2
  In1/1 -> Logical Operator/1, Logical Operator1/1
  Logical Operator1/1 -> Out1/1
  Logical Operator/1 -> Out2/1

== system Multiplier/8-Bit_Multiplier/Full adder38/Half adder1 ==
  In1 : Inport  OutDataTypeStr=boolean
  In2 : Inport  Port=2  OutDataTypeStr=boolean
  Logical Operator : Logic  AllPortsSameDT=off  OutDataTypeStr=boolean
  Logical Operator1 : Logic  Operator=XOR  AllPortsSameDT=off  OutDataTypeStr=boolean
  Out1 : Outport
  Out2 : Outport  Port=2
  wires:
  In2/1 -> Logical Operator/2, Logical Operator1/2
  In1/1 -> Logical Operator/1, Logical Operator1/1
  Logical Operator1/1 -> Out1/1
  Logical Operator/1 -> Out2/1

== system Multiplier/8-Bit_Multiplier/Full adder38/Half adder2 ==
  In1 : Inport  OutDataTypeStr=boolean
  In2 : Inport  Port=2  OutDataTypeStr=boolean
  Logical Operator : Logic  AllPortsSameDT=off  OutDataTypeStr=boolean
  Logical Operator1 : Logic  Operator=XOR  AllPortsSameDT=off  OutDataTypeStr=boolean
  Out1 : Outport
  Out2 : Outport  Port=2
  wires:
  In2/1 -> Logical Operator/2, Logical Operator1/2
  In1/1 -> Logical Operator/1, Logical Operator1/1
  Logical Operator1/1 -> Out1/1
  Logical Operator/1 -> Out2/1

== system Multiplier/8-Bit_Multiplier/Full adder39/Half adder1 ==
  In1 : Inport  OutDataTypeStr=boolean
  In2 : Inport  Port=2  OutDataTypeStr=boolean
  Logical Operator : Logic  AllPortsSameDT=off  OutDataTypeStr=boolean
  Logical Operator1 : Logic  Operator=XOR  AllPortsSameDT=off  OutDataTypeStr=boolean
  Out1 : Outport
  Out2 : Outport  Port=2
  wires:
  In2/1 -> Logical Operator/2, Logical Operator1/2
  In1/1 -> Logical Operator/1, Logical Operator1/1
  Logical Operator1/1 -> Out1/1
  Logical Operator/1 -> Out2/1

== system Multiplier/8-Bit_Multiplier/Full adder39/Half adder2 ==
  In1 : Inport  OutDataTypeStr=boolean
  In2 : Inport  Port=2  OutDataTypeStr=boolean
  Logical Operator : Logic  AllPortsSameDT=off  OutDataTypeStr=boolean
  Logical Operator1 : Logic  Operator=XOR  AllPortsSameDT=off  OutDataTypeStr=boolean
  Out1 : Outport
  Out2 : Outport  Port=2
  wires:
  In2/1 -> Logical Operator/2, Logical Operator1/2
  In1/1 -> Logical Operator/1, Logical Operator1/1
  Logical Operator1/1 -> Out1/1
  Logical Operator/1 -> Out2/1

== system Multiplier/8-Bit_Multiplier/Full adder4/Half adder1 ==
  In1 : Inport  OutDataTypeStr=boolean
  In2 : Inport  Port=2  OutDataTypeStr=boolean
  Logical Operator : Logic  AllPortsSameDT=off  OutDataTypeStr=boolean
  Logical Operator1 : Logic  Operator=XOR  AllPortsSameDT=off  OutDataTypeStr=boolean
  Out1 : Outport
  Out2 : Outport  Port=2
  wires:
  In2/1 -> Logical Operator/2, Logical Operator1/2
  In1/1 -> Logical Operator/1, Logical Operator1/1
  Logical Operator1/1 -> Out1/1
  Logical Operator/1 -> Out2/1

== system Multiplier/8-Bit_Multiplier/Full adder4/Half adder2 ==
  In1 : Inport  OutDataTypeStr=boolean
  In2 : Inport  Port=2  OutDataTypeStr=boolean
  Logical Operator : Logic  AllPortsSameDT=off  OutDataTypeStr=boolean
  Logical Operator1 : Logic  Operator=XOR  AllPortsSameDT=off  OutDataTypeStr=boolean
  Out1 : Outport
  Out2 : Outport  Port=2
  wires:
  In2/1 -> Logical Operator/2, Logical Operator1/2
  In1/1 -> Logical Operator/1, Logical Operator1/1
  Logical Operator1/1 -> Out1/1
  Logical Operator/1 -> Out2/1

== system Multiplier/8-Bit_Multiplier/Full adder40/Half adder1 ==
  In1 : Inport  OutDataTypeStr=boolean
  In2 : Inport  Port=2  OutDataTypeStr=boolean
  Logical Operator : Logic  AllPortsSameDT=off  OutDataTypeStr=boolean
  Logical Operator1 : Logic  Operator=XOR  AllPortsSameDT=off  OutDataTypeStr=boolean
  Out1 : Outport
  Out2 : Outport  Port=2
  wires:
  In2/1 -> Logical Operator/2, Logical Operator1/2
  In1/1 -> Logical Operator/1, Logical Operator1/1
  Logical Operator1/1 -> Out1/1
  Logical Operator/1 -> Out2/1

== system Multiplier/8-Bit_Multiplier/Full adder40/Half adder2 ==
  In1 : Inport  OutDataTypeStr=boolean
  In2 : Inport  Port=2  OutDataTypeStr=boolean
  Logical Operator : Logic  AllPortsSameDT=off  OutDataTypeStr=boolean
  Logical Operator1 : Logic  Operator=XOR  AllPortsSameDT=off  OutDataTypeStr=boolean
  Out1 : Outport
  Out2 : Outport  Port=2
  wires:
  In2/1 -> Logical Operator/2, Logical Operator1/2
  In1/1 -> Logical Operator/1, Logical Operator1/1
  Logical Operator1/1 -> Out1/1
  Logical Operator/1 -> Out2/1

== system Multiplier/8-Bit_Multiplier/Full adder41/Half adder1 ==
  In1 : Inport  OutDataTypeStr=boolean
  In2 : Inport  Port=2  OutDataTypeStr=boolean
  Logical Operator : Logic  AllPortsSameDT=off  OutDataTypeStr=boolean
  Logical Operator1 : Logic  Operator=XOR  AllPortsSameDT=off  OutDataTypeStr=boolean
  Out1 : Outport
  Out2 : Outport  Port=2
  wires:
  In2/1 -> Logical Operator/2, Logical Operator1/2
  In1/1 -> Logical Operator/1, Logical Operator1/1
  Logical Operator1/1 -> Out1/1
  Logical Operator/1 -> Out2/1

== system Multiplier/8-Bit_Multiplier/Full adder41/Half adder2 ==
  In1 : Inport  OutDataTypeStr=boolean
  In2 : Inport  Port=2  OutDataTypeStr=boolean
  Logical Operator : Logic  AllPortsSameDT=off  OutDataTypeStr=boolean
  Logical Operator1 : Logic  Operator=XOR  AllPortsSameDT=off  OutDataTypeStr=boolean
  Out1 : Outport
  Out2 : Outport  Port=2
  wires:
  In2/1 -> Logical Operator/2, Logical Operator1/2
  In1/1 -> Logical Operator/1, Logical Operator1/1
  Logical Operator1/1 -> Out1/1
  Logical Operator/1 -> Out2/1

== system Multiplier/8-Bit_Multiplier/Full adder42/Half adder1 ==
  In1 : Inport  OutDataTypeStr=boolean
  In2 : Inport  Port=2  OutDataTypeStr=boolean
  Logical Operator : Logic  AllPortsSameDT=off  OutDataTypeStr=boolean
  Logical Operator1 : Logic  Operator=XOR  AllPortsSameDT=off  OutDataTypeStr=boolean
  Out1 : Outport
  Out2 : Outport  Port=2
  wires:
  In2/1 -> Logical Operator/2, Logical Operator1/2
  In1/1 -> Logical Operator/1, Logical Operator1/1
  Logical Operator1/1 -> Out1/1
  Logical Operator/1 -> Out2/1

== system Multiplier/8-Bit_Multiplier/Full adder42/Half adder2 ==
  In1 : Inport  OutDataTypeStr=boolean
  In2 : Inport  Port=2  OutDataTypeStr=boolean
  Logical Operator : Logic  AllPortsSameDT=off  OutDataTypeStr=boolean
  Logical Operator1 : Logic  Operator=XOR  AllPortsSameDT=off  OutDataTypeStr=boolean
  Out1 : Outport
  Out2 : Outport  Port=2
  wires:
  In2/1 -> Logical Operator/2, Logical Operator1/2
  In1/1 -> Logical Operator/1, Logical Operator1/1
  Logical Operator1/1 -> Out1/1
  Logical Operator/1 -> Out2/1

== system Multiplier/8-Bit_Multiplier/Full adder43/Half adder1 ==
  In1 : Inport  OutDataTypeStr=boolean
  In2 : Inport  Port=2  OutDataTypeStr=boolean
  Logical Operator : Logic  AllPortsSameDT=off  OutDataTypeStr=boolean
  Logical Operator1 : Logic  Operator=XOR  AllPortsSameDT=off  OutDataTypeStr=boolean
  Out1 : Outport
  Out2 : Outport  Port=2
  wires:
  In2/1 -> Logical Operator/2, Logical Operator1/2
  In1/1 -> Logical Operator/1, Logical Operator1/1
  Logical Operator1/1 -> Out1/1
  Logical Operator/1 -> Out2/1

== system Multiplier/8-Bit_Multiplier/Full adder43/Half adder2 ==
  In1 : Inport  OutDataTypeStr=boolean
  In2 : Inport  Port=2  OutDataTypeStr=boolean
  Logical Operator : Logic  AllPortsSameDT=off  OutDataTypeStr=boolean
  Logical Operator1 : Logic  Operator=XOR  AllPortsSameDT=off  OutDataTypeStr=boolean
  Out1 : Outport
  Out2 : Outport  Port=2
  wires:
  In2/1 -> Logical Operator/2, Logical Operator1/2
  In1/1 -> Logical Operator/1, Logical Operator1/1
  Logical Operator1/1 -> Out1/1
  Logical Operator/1 -> Out2/1

== system Multiplier/8-Bit_Multiplier/Full adder44/Half adder1 ==
  In1 : Inport  OutDataTypeStr=boolean
  In2 : Inport  Port=2  OutDataTypeStr=boolean
  Logical Operator : Logic  AllPortsSameDT=off  OutDataTypeStr=boolean
  Logical Operator1 : Logic  Operator=XOR  AllPortsSameDT=off  OutDataTypeStr=boolean
  Out1 : Outport
  Out2 : Outport  Port=2
  wires:
  In2/1 -> Logical Operator/2, Logical Operator1/2
  In1/1 -> Logical Operator/1, Logical Operator1/1
  Logical Operator1/1 -> Out1/1
  Logical Operator/1 -> Out2/1

== system Multiplier/8-Bit_Multiplier/Full adder44/Half adder2 ==
  In1 : Inport  OutDataTypeStr=boolean
  In2 : Inport  Port=2  OutDataTypeStr=boolean
  Logical Operator : Logic  AllPortsSameDT=off  OutDataTypeStr=boolean
  Logical Operator1 : Logic  Operator=XOR  AllPortsSameDT=off  OutDataTypeStr=boolean
  Out1 : Outport
  Out2 : Outport  Port=2
  wires:
  In2/1 -> Logical Operator/2, Logical Operator1/2
  In1/1 -> Logical Operator/1, Logical Operator1/1
  Logical Operator1/1 -> Out1/1
  Logical Operator/1 -> Out2/1

== system Multiplier/8-Bit_Multiplier/Full adder45/Half adder1 ==
  In1 : Inport  OutDataTypeStr=boolean
  In2 : Inport  Port=2  OutDataTypeStr=boolean
  Logical Operator : Logic  AllPortsSameDT=off  OutDataTypeStr=boolean
  Logical Operator1 : Logic  Operator=XOR  AllPortsSameDT=off  OutDataTypeStr=boolean
  Out1 : Outport
  Out2 : Outport  Port=2
  wires:
  In2/1 -> Logical Operator/2, Logical Operator1/2
  In1/1 -> Logical Operator/1, Logical Operator1/1
  Logical Operator1/1 -> Out1/1
  Logical Operator/1 -> Out2/1

== system Multiplier/8-Bit_Multiplier/Full adder45/Half adder2 ==
  In1 : Inport  OutDataTypeStr=boolean
  In2 : Inport  Port=2  OutDataTypeStr=boolean
  Logical Operator : Logic  AllPortsSameDT=off  OutDataTypeStr=boolean
  Logical Operator1 : Logic  Operator=XOR  AllPortsSameDT=off  OutDataTypeStr=boolean
  Out1 : Outport
  Out2 : Outport  Port=2
  wires:
  In2/1 -> Logical Operator/2, Logical Operator1/2
  In1/1 -> Logical Operator/1, Logical Operator1/1
  Logical Operator1/1 -> Out1/1
  Logical Operator/1 -> Out2/1

== system Multiplier/8-Bit_Multiplier/Full adder46/Half adder1 ==
  In1 : Inport  OutDataTypeStr=boolean
  In2 : Inport  Port=2  OutDataTypeStr=boolean
  Logical Operator : Logic  AllPortsSameDT=off  OutDataTypeStr=boolean
  Logical Operator1 : Logic  Operator=XOR  AllPortsSameDT=off  OutDataTypeStr=boolean
  Out1 : Outport
  Out2 : Outport  Port=2
  wires:
  In2/1 -> Logical Operator/2, Logical Operator1/2
  In1/1 -> Logical Operator/1, Logical Operator1/1
  Logical Operator1/1 -> Out1/1
  Logical Operator/1 -> Out2/1

== system Multiplier/8-Bit_Multiplier/Full adder46/Half adder2 ==
  In1 : Inport  OutDataTypeStr=boolean
  In2 : Inport  Port=2  OutDataTypeStr=boolean
  Logical Operator : Logic  AllPortsSameDT=off  OutDataTypeStr=boolean
  Logical Operator1 : Logic  Operator=XOR  AllPortsSameDT=off  OutDataTypeStr=boolean
  Out1 : Outport
  Out2 : Outport  Port=2
  wires:
  In2/1 -> Logical Operator/2, Logical Operator1/2
  In1/1 -> Logical Operator/1, Logical Operator1/1
  Logical Operator1/1 -> Out1/1
  Logical Operator/1 -> Out2/1

== system Multiplier/8-Bit_Multiplier/Full adder47/Half adder1 ==
  In1 : Inport  OutDataTypeStr=boolean
  In2 : Inport  Port=2  OutDataTypeStr=boolean
  Logical Operator : Logic  AllPortsSameDT=off  OutDataTypeStr=boolean
  Logical Operator1 : Logic  Operator=XOR  AllPortsSameDT=off  OutDataTypeStr=boolean
  Out1 : Outport
  Out2 : Outport  Port=2
  wires:
  In2/1 -> Logical Operator/2, Logical Operator1/2
  In1/1 -> Logical Operator/1, Logical Operator1/1
  Logical Operator1/1 -> Out1/1
  Logical Operator/1 -> Out2/1

== system Multiplier/8-Bit_Multiplier/Full adder47/Half adder2 ==
  In1 : Inport  OutDataTypeStr=boolean
  In2 : Inport  Port=2  OutDataTypeStr=boolean
  Logical Operator : Logic  AllPortsSameDT=off  OutDataTypeStr=boolean
  Logical Operator1 : Logic  Operator=XOR  AllPortsSameDT=off  OutDataTypeStr=boolean
  Out1 : Outport
  Out2 : Outport  Port=2
  wires:
  In2/1 -> Logical Operator/2, Logical Operator1/2
  In1/1 -> Logical Operator/1, Logical Operator1/1
  Logical Operator1/1 -> Out1/1
  Logical Operator/1 -> Out2/1

== system Multiplier/8-Bit_Multiplier/Full adder48/Half adder1 ==
  In1 : Inport  OutDataTypeStr=boolean
  In2 : Inport  Port=2  OutDataTypeStr=boolean
  Logical Operator : Logic  AllPortsSameDT=off  OutDataTypeStr=boolean
  Logical Operator1 : Logic  Operator=XOR  AllPortsSameDT=off  OutDataTypeStr=boolean
  Out1 : Outport
  Out2 : Outport  Port=2
  wires:
  In2/1 -> Logical Operator/2, Logical Operator1/2
  In1/1 -> Logical Operator/1, Logical Operator1/1
  Logical Operator1/1 -> Out1/1
  Logical Operator/1 -> Out2/1

== system Multiplier/8-Bit_Multiplier/Full adder48/Half adder2 ==
  In1 : Inport  OutDataTypeStr=boolean
  In2 : Inport  Port=2  OutDataTypeStr=boolean
  Logical Operator : Logic  AllPortsSameDT=off  OutDataTypeStr=boolean
  Logical Operator1 : Logic  Operator=XOR  AllPortsSameDT=off  OutDataTypeStr=boolean
  Out1 : Outport
  Out2 : Outport  Port=2
  wires:
  In2/1 -> Logical Operator/2, Logical Operator1/2
  In1/1 -> Logical Operator/1, Logical Operator1/1
  Logical Operator1/1 -> Out1/1
  Logical Operator/1 -> Out2/1

== system Multiplier/8-Bit_Multiplier/Full adder5/Half adder1 ==
  In1 : Inport  OutDataTypeStr=boolean
  In2 : Inport  Port=2  OutDataTypeStr=boolean
  Logical Operator : Logic  AllPortsSameDT=off  OutDataTypeStr=boolean
  Logical Operator1 : Logic  Operator=XOR  AllPortsSameDT=off  OutDataTypeStr=boolean
  Out1 : Outport
  Out2 : Outport  Port=2
  wires:
  In2/1 -> Logical Operator/2, Logical Operator1/2
  In1/1 -> Logical Operator/1, Logical Operator1/1
  Logical Operator1/1 -> Out1/1
  Logical Operator/1 -> Out2/1

== system Multiplier/8-Bit_Multiplier/Full adder5/Half adder2 ==
  In1 : Inport  OutDataTypeStr=boolean
  In2 : Inport  Port=2  OutDataTypeStr=boolean
  Logical Operator : Logic  AllPortsSameDT=off  OutDataTypeStr=boolean
  Logical Operator1 : Logic  Operator=XOR  AllPortsSameDT=off  OutDataTypeStr=boolean
  Out1 : Outport
  Out2 : Outport  Port=2
  wires:
  In2/1 -> Logical Operator/2, Logical Operator1/2
  In1/1 -> Logical Operator/1, Logical Operator1/1
  Logical Operator1/1 -> Out1/1
  Logical Operator/1 -> Out2/1

== system Multiplier/8-Bit_Multiplier/Full adder6/Half adder1 ==
  In1 : Inport  OutDataTypeStr=boolean
  In2 : Inport  Port=2  OutDataTypeStr=boolean
  Logical Operator : Logic  AllPortsSameDT=off  OutDataTypeStr=boolean
  Logical Operator1 : Logic  Operator=XOR  AllPortsSameDT=off  OutDataTypeStr=boolean
  Out1 : Outport
  Out2 : Outport  Port=2
  wires:
  In2/1 -> Logical Operator/2, Logical Operator1/2
  In1/1 -> Logical Operator/1, Logical Operator1/1
  Logical Operator1/1 -> Out1/1
  Logical Operator/1 -> Out2/1

== system Multiplier/8-Bit_Multiplier/Full adder6/Half adder2 ==
  In1 : Inport  OutDataTypeStr=boolean
  In2 : Inport  Port=2  OutDataTypeStr=boolean
  Logical Operator : Logic  AllPortsSameDT=off  OutDataTypeStr=boolean
  Logical Operator1 : Logic  Operator=XOR  AllPortsSameDT=off  OutDataTypeStr=boolean
  Out1 : Outport
  Out2 : Outport  Port=2
  wires:
  In2/1 -> Logical Operator/2, Logical Operator1/2
  In1/1 -> Logical Operator/1, Logical Operator1/1
  Logical Operator1/1 -> Out1/1
  Logical Operator/1 -> Out2/1
